simulink model "Lamp_SF"  (R2018b)
settings: Solver=FixedStepDiscrete  StartTime=0.0  StopTime=50  RelTol=1e-3
settings Model: Creator=lenovo2  LastModifiedBy=mostafa
settings OptimizationCC: DefaultParameterBehavior=Inlined  EnhancedBackFolding=on  PassReuseOutputArgsAs=Individual arguments  OptimizeBlockOrder=speed  DifferentSizesBufferReuse=on  OptimizationCustomize=off
settings DebuggingCC: UnderspecifiedInitializationDetection=Classic  MergeDetectMultiDrivingBlocksExec=none  ParameterTunabilityLossMsg=error
settings ModelReferenceCC: PropagateSignalLabelsOutOfModel=off
settings SFSimCC: MATLABDynamicMemAlloc=off
settings RTWCC: SystemTargetFile=ert.tlc  GenCodeOnly=on  TemplateMakefile=ert_default_tmf  GenerateReport=on  IncludeHyperlinkInReport=on  LaunchReport=on  GenerateTraceInfo=on  GenerateTraceReport=on  GenerateTraceReportSl=on  GenerateTraceReportSf=on  GenerateTraceReportEml=on
settings CodeAppCC: ForceParamTrailComments=on  IgnoreCustomStorageClasses=off  OperatorAnnotations=on  SimulinkDataObjDesc=on  SFDataObjDesc=on  InsertBlockDesc=on
settings ERTTargetCC: TargetLangStandard=C99 (ISO)  GenerateSampleERTMain=on  InlinedParameterPlacement=NonHierarchical  ERTCustomFileTemplate=example_file_process.tlc

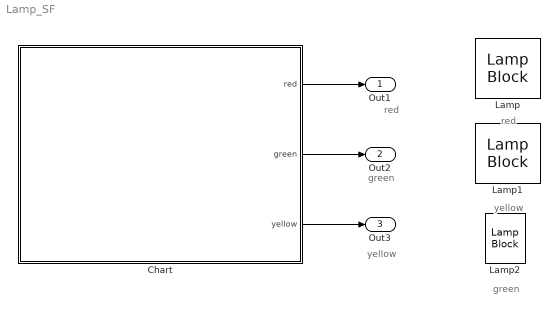
== system Lamp_SF ==
  note: red
  note: green
  note: yellow
  note: green
  note: yellow
  note: red
  Chart : Stateflow chart  TreatAsAtomicUnit=on
  Lamp : LampBlock  WebBlockId=2
  Lamp1 : LampBlock  WebBlockId=3
  Lamp2 : LampBlock  WebBlockId=4
  Out1 : Outport
  Out2 : Outport  Port=2
  Out3 : Outport  Port=3
  wires:
  Chart/1(red) -> Out1/1
  Chart/3(yellow) -> Out3/1
  Chart/2(green) -> Out2/1

== stateflow chart Lamp_SF/Chart ==
  state Green
    en:
    red=0;
    yellow=0;
    green=0;
    du:
    red = 0;
    green=1;
    yellow=0;
    after(3,sec);
    green=0;
    ex:
    green=0;
  state Yellow
    en:
    red=0;
    yellow=0;
    green=0;
    du:
    red = 0;
    green=0;
    yellow=1;
    after(3,sec);
    ex:
    yellow=0;
  state Red
    en:
    du:
    red = 1;
    green=0;
    yellow=0;
    [after(5,sec)]
    ex:
    red=0;
  (default) -> Red
  Red -> Yellow
  Yellow -> Green : [after(3,sec)]
  Green -> Red : [after(5,sec)]
  data: red output uint8 =uint8(0); green output uint8 =uint8(0); yellow output uint8 =uint8(0)
